simulink model "mass_spring_damper"  (R2022a)
settings: Solver=VariableStepAuto  StartTime=0.0  StopTime=10.0  MaxStep=1e-2  RelTol=1e-3
InitFcn:
  | start;
values from neighbouring files (symbols this model uses):
  d = 1    [start.m]
  dy0 = 0    [start.m]
  F_ext = 1    [start.m]
  k = 2    [start.m]
  m = 1    [start.m]
  y0 = 0    [start.m]
settings Model: Creator=mathe  LastModifiedBy=mathe

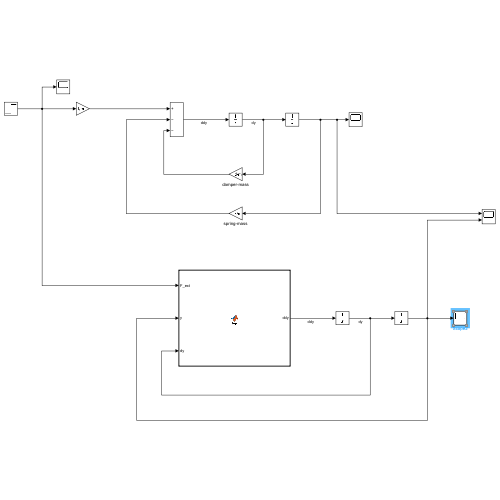
[thumbnail: Simulink's stored preview of the top-level diagram]
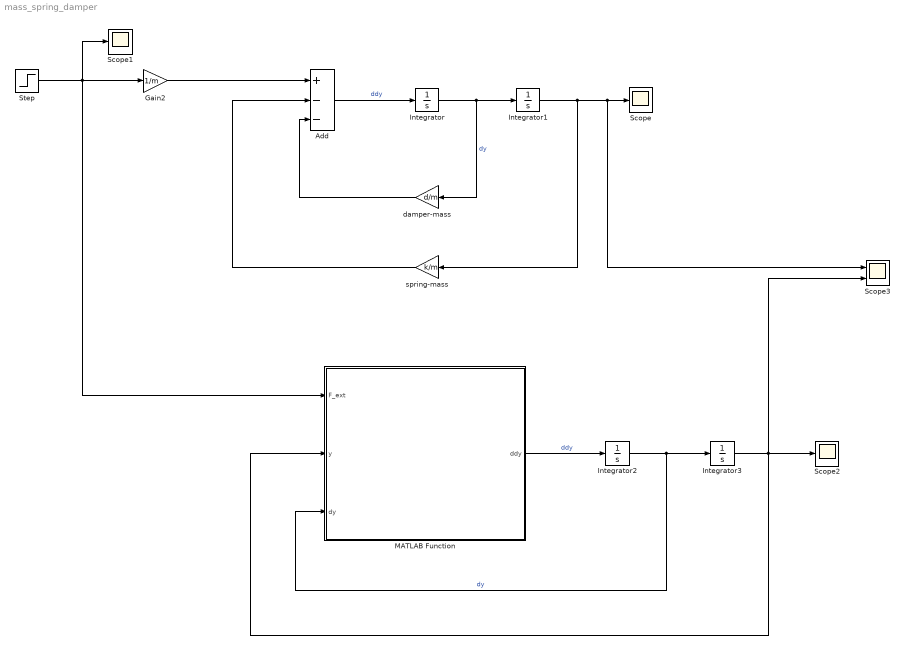
== system mass_spring_damper ==
  Add : Sum  Inputs=+--
  Gain2 : Gain  Gain=1/m
  Integrator : Integrator  InitialCondition=dy0
  Integrator1 : Integrator  InitialCondition=y0
  Integrator2 : Integrator  InitialCondition=dy0
  Integrator3 : Integrator  InitialCondition=y0
  MATLAB Function : MATLAB Function  TreatAsAtomicUnit=on
  Scope : Scope
  Scope1 : Scope
  Scope2 : Scope
  Scope3 : Scope  NumInputPorts=2
  Step : Step  After=F_ext  SampleTime=0
  damper-mass : Gain  Gain=d/m
  spring-mass : Gain  Gain=k/m
  wires:
  Integrator/1 -> damper-mass/1, Integrator1/1  "dy"
  Add/1 -> Integrator/1  "ddy"
  damper-mass/1 -> Add/3
  Integrator1/1 -> Scope3/1, Scope/1, spring-mass/1
  spring-mass/1 -> Add/2
  Gain2/1 -> Add/1
  Step/1 -> MATLAB Function/1(F_ext), Scope1/1, Gain2/1
  Integrator2/1 -> Integrator3/1, MATLAB Function/3(dy)  "dy"
  MATLAB Function/1(ddy) -> Integrator2/1  "ddy"
  Integrator3/1 -> Scope3/2, Scope2/1, MATLAB Function/2(y)

== matlab function mass_spring_damper/MATLAB Function ==
  data: F_ext input; ddy output; y input; dy input; m parameter; k parameter; d parameter
function ddy = fcn(F_ext, y, dy, m, k, d)

ddy = F_ext/m - d/m*dy - k/m*y;
